simulink model "vC_1ph_MR2"  (Simulink 7.9)
settings: Solver=ode14x  StartTime=0.0  StopTime=20/60  FixedStep=Ts1  RelTol=1e-3
PostLoadFcn:
  | , if any(exist('dsrtsu_mdlpostloadfcn', 'file') == [2, 3, 6]), try dsrtsu_mdlpostloadfcn('Execute', bdroot); catch fprintf('Error in PostLoadFcn (dsrtsu_mdlpostloadfcn) for model "%s":\n %s\n', bdroot, lasterr); end, end,
InitFcn:
  | vC_ini
values from neighbouring files (symbols this model uses):
  C = Cideal+deltaC    (= 4e-05)    [IMC_calculo_limites_thetas.m]    (also in IMC_ini.m; JORGE_controlador_LCL_malha_interna.m; LCL_PAPM.m; R_in_LCL.m)
  excitacao_persistente = 0    [iC_ini.m]    (also in vC_ini.m)
  init_time = 20000/60    (= 333.333333333)    [iC_ini.m]    (also in vC_ini.m)
  L1 = L1ideal+deltaL1    (= 0.002)    [IMC_calculo_limites_thetas.m]    (also in IMC_ini.m; LCL_PAPM.m; R_in_LCL.m; calculo_FTs.m)
  L2 = L2ideal+deltaL2+Lgideal+deltaLg    (= 0.002)    [IMC_calculo_limites_thetas.m]    (also in IMC_ini.m; LCL_PAPM.m; R_in_LCL.m; calculo_FTs.m)
  param_change_time = 20000/60    (= 333.333333333)    [iC_ini.m]    (also in vC_ini.m)
  R1 = R1ideal+deltaR1    (= 1)    [IMC_calculo_limites_thetas.m]    (also in IMC_ini.m; R_in_LCL.m = 0; gera_resultados.m = 0; iC_ini.m = 0)
  R2 = R2ideal+deltaR2+Rgideal+deltaRg    (= 1)    [IMC_calculo_limites_thetas.m]    (also in IMC_ini.m; R_in_LCL.m = 0; gera_resultados.m = 0; iC_ini.m = 0)
  R_init = 10    [iC_ini.m]    (also in vC_ini.m)
  rede_amp = 311    [iC_ini.m]    (also in vC_ini.m)
  ref_amp = 10    [iC_ini.m]    (also in vC_ini.m = 200)
  ref_amp11 = ref_amp/2    (= 5)    [iC_ini.m]    (also in vC_ini.m = 100)
  ref_amp13 = ref_amp/2    (= 5)    [iC_ini.m]    (also in vC_ini.m = 100)
  ref_amp3 = ref_amp/2    (= 5)    [iC_ini.m]    (also in vC_ini.m = 100)
  ref_amp5 = ref_amp/2    (= 5)    [iC_ini.m]    (also in vC_ini.m = 100)
  ref_amp7 = ref_amp/2    (= 5)    [iC_ini.m]    (also in vC_ini.m = 100)
  ref_amp9 = ref_amp/2    (= 5)    [iC_ini.m]    (also in vC_ini.m = 100)
  ref_freq = 2*pi*60    (= 376.991118431)    [iC_ini.m]    (also in vC_ini.m)
  ref_phaseInv_time = 20000/60    (= 333.333333333)    [iC_ini.m]    (also in vC_ini.m)
  ref_step_time = 20000/60    (= 333.333333333)    [iC_ini.m]    (also in vC_ini.m)
  Ts = 0.5    [IMC_calculo_limites_thetas.m]    (also in IMC_datta_ini.m; IMC_ini.m = 8.33333333333e-05; JORGE_controlador_LCL_malha_interna.m = 8.33333333333e-05; LCL_PAPM.m = 8.33333333333e-05)
  Ts1 = Ts/10    (= 8.33333333333e-06)    [iC_ini.m]    (also in vC_ini.m)
  VCC = 400    [iC_ini.m]    (also in vC_ini.m)
libraries: powerlib x15, powerlib_extras x1
settings Model: DSRTSU_INTERNAL_RTI_VER=390  DSRTSU_INTERNAL_RTI_TYPE=rti1103  Creator=dpbernardon  LastModifiedBy=marcelodurgante  BufferReuse=off
settings SolverCC: AutoInsertRateTranBlk=on
settings OptimizationCC: BlockReduction=off  OptimizeBlockIOStorage=off  BufferReuse=off  ExpressionFolding=off  LocalBlockOutputs=off
settings DebuggingCC: FcnCallInpInsideContextMsg=Use local settings  UnconnectedInputMsg=none  UnconnectedOutputMsg=none  UnconnectedLineMsg=none
settings HardwareCC: ProdIntDivRoundTo=Zero  ProdEndianess=BigEndian  ProdHWDeviceType=Generic->Custom  TargetIntDivRoundTo=Zero  TargetEndianess=BigEndian  TargetHWDeviceType=Generic->Custom
settings RTWCC: SystemTargetFile=rti1103.tlc  MakeCommand=make_rti  TemplateMakefile=rti1103.tmf  Description=dSPACE DS1103 Hardware Platform  ProcessScript=rti1103_make_rtw_hook
settings STFCustomTargetCC: CodeReplacementLibrary=ANSI_C  ParMdlRefBuildCompliant=on  GeneratePreprocessorConditionals=Disable all  MatFileLogging=on  SystemTargetFile=rti1103.tlc
settings GRTTargetCC: CompOptLevelCompliant=off  ConcurrentExecutionCompliant=off  CombineOutputUpdateFcns=off  GRTInterface=on  ExtModeMexFile=noextcomm
settings CustomProperty: DataType=RTWOptions_EnumType_C__dSPACE RCPHIL 72_matlab_rti1103_tlc_rti1103_1InitialSimState  Value=RUN
settings EnumStrPairs: String=RUN

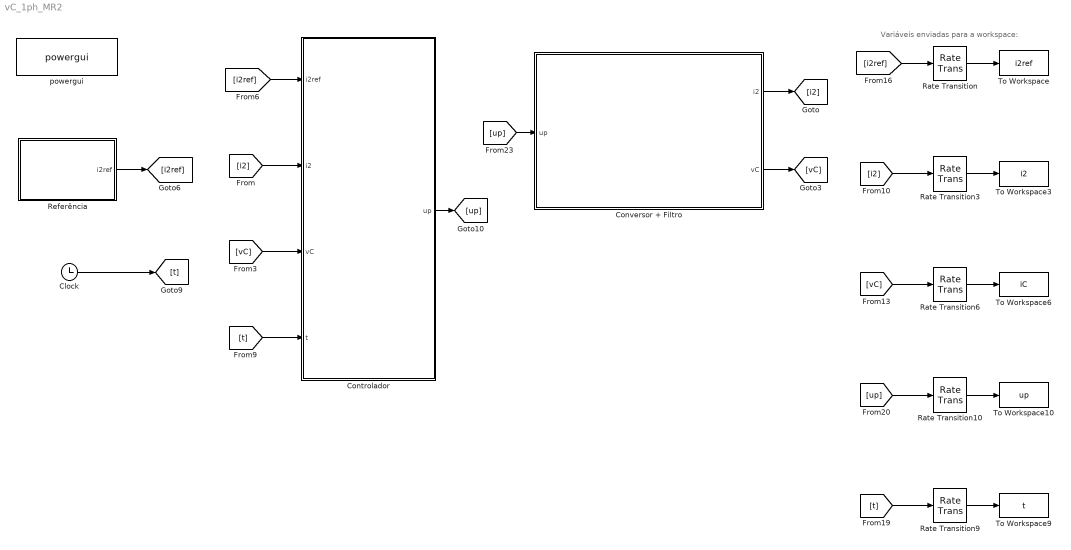
== system vC_1ph_MR2 ==
  note: Variáveis enviadas para a workspace:
  Clock : Clock
  Controlador : Subsystem
  Conversor + Filtro : Subsystem
  Rate Transition{,3,6,9..10} (5 alike) : RateTransition  OutPortSampleTime=Ts1
  Referência : Subsystem
  To Workspace : ToWorkspace  VariableName=i2ref  SampleTime=Ts1
  To Workspace10 : ToWorkspace  VariableName=up  SampleTime=Ts1
  To Workspace3 : ToWorkspace  VariableName=i2  SampleTime=Ts1
  To Workspace6 : ToWorkspace  VariableName=iC  SampleTime=Ts1
  To Workspace9 : ToWorkspace  VariableName=t  SampleTime=Ts1
  powergui : powerlib/powergui  Priority=1  SimulationMode=Discrete  SolverType=Tustin  SampleTime=Ts1  frequency=60  SPID=off  DisableSnubberDevices=off  DisableRonSwitches=off  DisableVfSwitches=off  SwTol=0  Interpol=off  DisplayEquations=off  FunctionMessages=off  frequencyindice=0  Pbase=100e6  ErrMax=1e-4  Iterations=50  UnitsV=kV  UnitsW=MW  echomessages=off  HookPort=off  EnableUseOfTLC=off  x0status=blocks  RestoreLinks=warning  ResistiveCurrentMeasurement=off  Frange=[0:2:500]  Ylog=off  Xlog=on  ShowGrid=off  save=off  variable=ZData  ZoomFFT=off  StartTime=0.0  cycles=1  DisplayStyle=1  fundamental=60  FreqAxis=off  MaxFrequency=1000  frequencyindicesteady=1  RmsSteady=1  display=off  Ts=0  methode=off
  wires:
  Conversor + Filtro/1(i2) -> [i2]
  Conversor + Filtro/2(vC) -> [vC]
  [i2] -> Controlador/2(i2)
  [vC] -> Controlador/3(vC)
  Referência/1(i2ref) -> [i2ref]
  [i2ref] -> Controlador/1(i2ref)
  Clock/1 -> [t]
  [t] -> Controlador/4(t)
  [i2ref] -> Rate Transition/1
  [i2] -> Rate Transition3/1
  [vC] -> Rate Transition6/1
  [t] -> Rate Transition9/1
  Rate Transition/1 -> To Workspace/1
  Rate Transition3/1 -> To Workspace3/1
  Rate Transition6/1 -> To Workspace6/1
  Rate Transition9/1 -> To Workspace9/1
  [up] -> Rate Transition10/1
  Rate Transition10/1 -> To Workspace10/1
  Controlador/1(up) -> [up]
  [up] -> Conversor + Filtro/1(up)

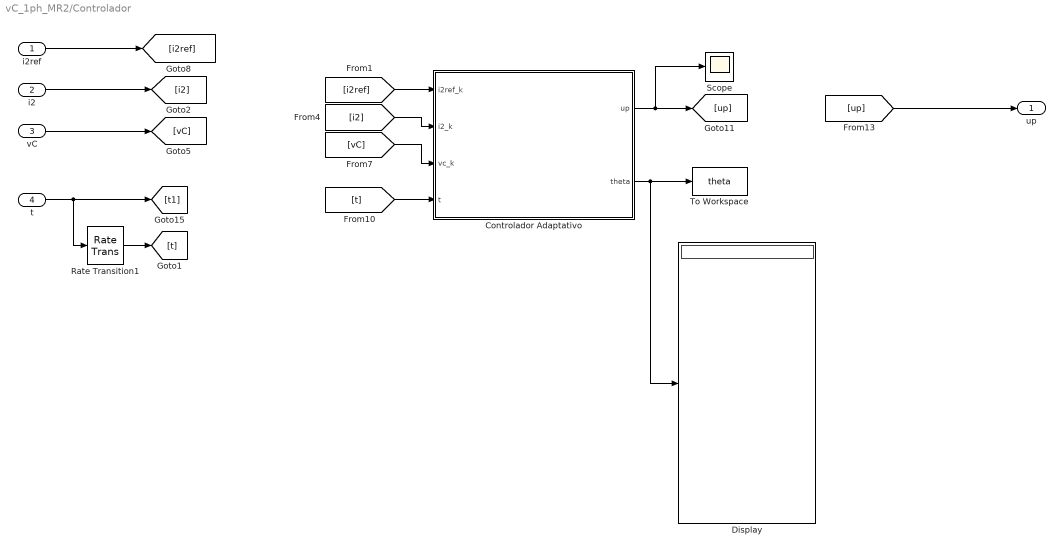
== system vC_1ph_MR2/Controlador ==
  i2ref : Inport
  i2 : Inport  Port=2
  vC : Inport  Port=3
  t : Inport  Port=4
  Controlador Adaptativo : MATLAB Function  TreatAsAtomicUnit=on  SystemSampleTime=Ts
      settings: MinAlgLoopOccurrences=on  RTWSystemCode=Function
  Display : Display
  Rate Transition1 : RateTransition  OutPortSampleTime=Ts
  Scope : Scope
      settings: YMin=-5500  YMax=5000  SaveName=ScopeData4
  To Workspace : ToWorkspace  VariableName=theta  SampleTime=Ts1
  up : Outport
  wires:
  t/1 -> Rate Transition1/1, [t1]
  Rate Transition1/1 -> [t]
  i2/1 -> [i2]
  vC/1 -> [vC]
  [i2ref] -> Controlador Adaptativo/1(i2ref_k)
  [i2] -> Controlador Adaptativo/2(i2_k)
  [vC] -> Controlador Adaptativo/3(vc_k)
  [up] -> up/1
  Controlador Adaptativo/2(theta) -> To Workspace/1, Display/1
  i2ref/1 -> [i2ref]
  Controlador Adaptativo/1(up) -> [up], Scope/1
  [t] -> Controlador Adaptativo/4(t)

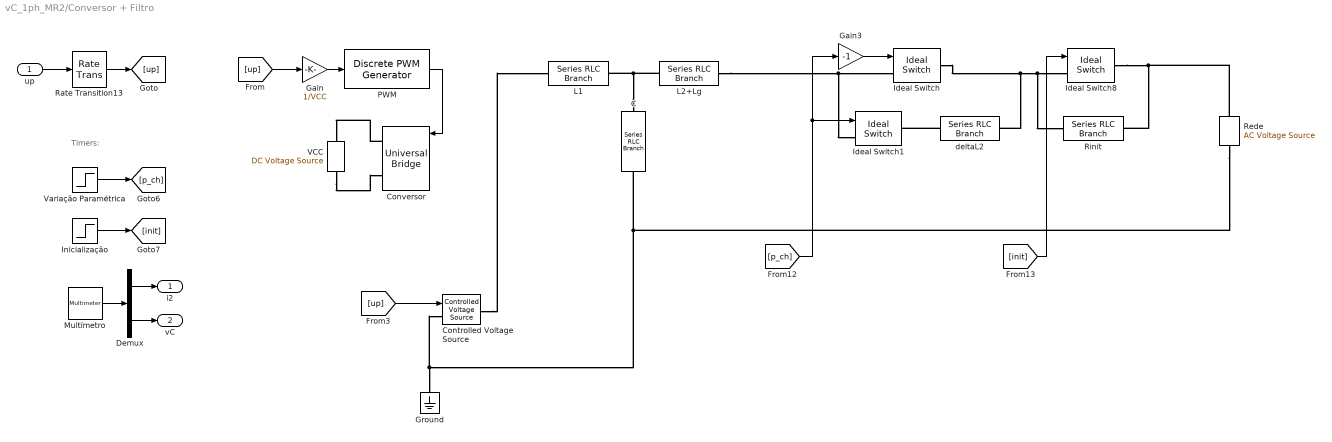
== system vC_1ph_MR2/Conversor + Filtro ==
  note: Timers:
  up : Inport
  C : powerlib/Elements/Series RLC Branch  LConnTagsString=__new0  RConnTagsString=__new0  BranchType=C  Resistance=1  Inductance=1e-3  SetiL0=off  InitialCurrent=0  Capacitance=C  Setx0=off  InitialVoltage=0  Measurements=Branch voltage
  Controlled Voltage Source : powerlib/Electrical Sources/Controlled Voltage Source  Initialize=on  Source_Type=AC  Amplitude=0  Phase=0  Frequency=0  Measurements=None
  Conversor : powerlib/Power Electronics/Universal Bridge  Arms=3  SnubberResistance=1e5  SnubberCapacitance=inf  Device=IGBT / Diodes  Ron=1e-3  Lon=0  ForwardVoltages="[  0  0  ]"  ForwardVoltage=0  GTOparameters=[ 10e-6 , 20e-6 ]  IGBTparameters=[ 1e-6 , 2e-6 ]  Measurements=UAB UBC UCA UDC voltages  Measurements_2=None  converterType=Rectifier
  Demux : Demux  Outputs=2
  Gain : Gain  Gain=1/VCC  SampleTime=Ts1
  Gain3 : Gain  Gain=-1  SampleTime=Ts1
  Ground : powerlib/Elements/Ground  LConnTagsString=a
  Ideal Switch : powerlib/Power Electronics/Ideal Switch  Ron=0.001  Lon=0  IC=1  Rs=1e5  Cs=inf  Measurements=off
  Ideal Switch1 : powerlib/Power Electronics/Ideal Switch  Ron=0.001  Lon=0  IC=0  Rs=1e5  Cs=inf  Measurements=off
  Ideal Switch8 : powerlib/Power Electronics/Ideal Switch  Ron=0.001  Lon=0  IC=1  Rs=1e5  Cs=inf  Measurements=off
  Inicialização : Step  Time=init_time  Before=1  After=0  SampleTime=Ts1
  L1 : powerlib/Elements/Series RLC Branch  LConnTagsString=__new0  RConnTagsString=__new0  BranchType=RL  Resistance=R1  Inductance=L1  SetiL0=off  InitialCurrent=0  Capacitance=1e-6  Setx0=off  InitialVoltage=0  Measurements=None
  L2+Lg : powerlib/Elements/Series RLC Branch  LConnTagsString=__new0  RConnTagsString=__new0  BranchType=RL  Resistance=R2  Inductance=L2  SetiL0=off  InitialCurrent=0  Capacitance=1e-6  Setx0=off  InitialVoltage=0  Measurements=Branch current
  Multímetro : powerlib/Measurements/Multimeter  PhasorSimulation=off  OutputType=Complex  sel=[6 1]  L=6  Gain=[1 1]  yselected={'Ib: Conversor + Filtro/L2+Lg','Ub: Conversor + Filtro/C'};  PSBOutputType=1  PSBequivalent=0  AxesSetting=[0,0.1,-100,100]  Display=0  SavedBlockNames=-11
  PWM : powerlib_extras/Discrete  Control Blocks/Discrete PWM Generator  GeneratorMode="3-arm  bridge (6 pulses)"  Fc=12000  Ts=Ts1  Internal=off  mIndex=0.4  Freq=60  Phase=0
  Rate Transition13 : RateTransition  OutPortSampleTime=Ts1
  Rede : powerlib/Electrical Sources/AC Voltage Source  Amplitude=rede_amp  Phase=0  Frequency=60  SampleTime=0  Measurements=None
  Rinit : powerlib/Elements/Series RLC Branch  LConnTagsString=__new0  RConnTagsString=__new0  BranchType=RL  Resistance=R_init  Inductance=5*L2  SetiL0=off  InitialCurrent=0  Capacitance=1e-6  Setx0=off  InitialVoltage=0  Measurements=None
  VCC : powerlib/Electrical Sources/DC Voltage Source  Amplitude=VCC  Measurements=None
  Variação Paramétrica : Step  Time=param_change_time  Before=-1  SampleTime=Ts1
  deltaL2 : powerlib/Elements/Series RLC Branch  LConnTagsString=__new0  RConnTagsString=__new0  BranchType=RL  Resistance=0  Inductance=5*L2  SetiL0=off  InitialCurrent=0  Capacitance=1e-6  Setx0=off  InitialVoltage=0  Measurements=None
  i2 : Outport
  vC : Outport  Port=2
  wires:
  Gain/1 -> PWM/1
  up/1 -> Rate Transition13/1
  Rate Transition13/1 -> [up]
  PWM/1 -> Conversor/1
  [up] -> Gain/1
  [up] -> Controlled Voltage Source/1
  Multímetro/1 -> Demux/1
  Demux/1 -> i2/1
  Variação Paramétrica/1 -> [p_ch]
  Gain3/1 -> Ideal Switch/1
  [init] -> Ideal Switch8/1
  Inicialização/1 -> [init]
  [p_ch] -> Gain3/1, Ideal Switch1/1
  Demux/2 -> vC/1
  connections:
  Ideal Switch/RConn1 -- deltaL2/RConn1 -- Ideal Switch8/LConn1 -- Rinit/LConn1
  C/LConn1 -- L2+Lg/LConn1 -- L1/RConn1
  Conversor/RConn1 -- VCC/RConn1
  VCC/LConn1 -- Conversor/RConn2
  L2+Lg/RConn1 -- Ideal Switch/LConn1 -- Ideal Switch1/LConn1
  deltaL2/LConn1 -- Ideal Switch1/RConn1
  Controlled Voltage Source/RConn1 -- L1/LConn1
  Rede/RConn1 -- Ideal Switch8/RConn1 -- Rinit/RConn1
  Controlled Voltage Source/LConn1 -- Ground/LConn1 -- C/RConn1 -- Rede/LConn1

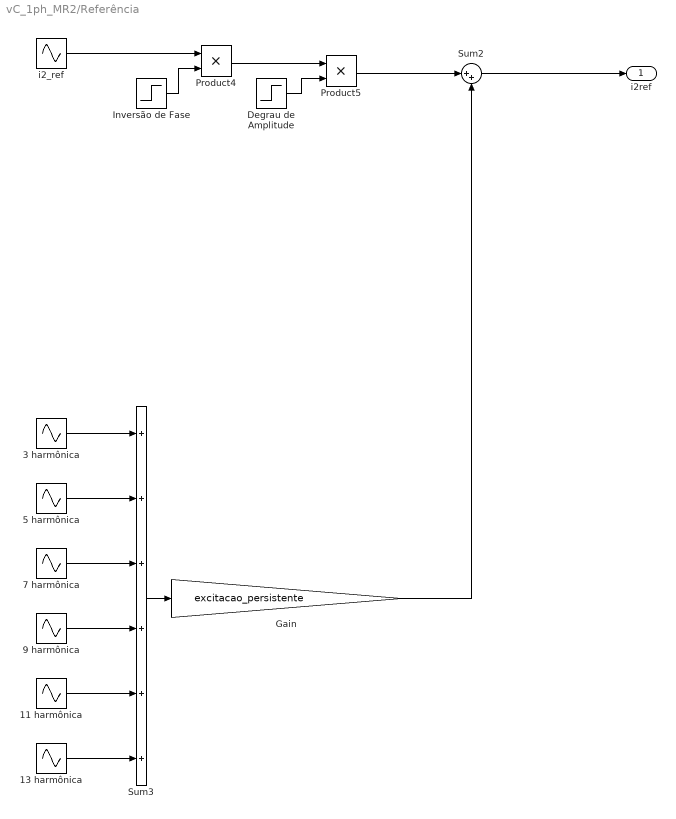
== system vC_1ph_MR2/Referência ==
  11 harmônica : Sin  Amplitude=ref_amp11  Frequency=ref_freq*11  SampleTime=Ts
  13 harmônica : Sin  Amplitude=ref_amp13  Frequency=ref_freq*13  SampleTime=Ts
  3 harmônica : Sin  Amplitude=ref_amp3  Frequency=ref_freq*3  SampleTime=Ts
  5 harmônica : Sin  Amplitude=ref_amp5  Frequency=ref_freq*5  SampleTime=Ts
  7 harmônica : Sin  Amplitude=ref_amp7  Frequency=ref_freq*7  SampleTime=Ts
  9 harmônica : Sin  Amplitude=ref_amp9  Frequency=ref_freq*9  SampleTime=Ts
  Degrau de Amplitude : Step  Time=ref_step_time  Before=1  After=2  SampleTime=Ts
  Gain : Gain  Gain=excitacao_persistente  SampleTime=Ts
  Inversão de Fase : Step  Time=ref_phaseInv_time  Before=1  After=-1  SampleTime=Ts
  Product4 : Product  SampleTime=Ts  RndMeth=Zero
  Product5 : Product  SampleTime=Ts  RndMeth=Zero
  Sum2 : Sum  Inputs=|++
  Sum3 : Sum  Inputs=++++++
  i2_ref : Sin  Amplitude=ref_amp  Frequency=ref_freq  SampleTime=Ts
  i2ref : Outport
  wires:
  Product4/1 -> Product5/1
  Inversão de Fase/1 -> Product4/2
  Degrau de Amplitude/1 -> Product5/2
  i2_ref/1 -> Product4/1
  Product5/1 -> Sum2/1
  Gain/1 -> Sum2/2
  Sum2/1 -> i2ref/1
  3 harmônica/1 -> Sum3/1
  5 harmônica/1 -> Sum3/2
  7 harmônica/1 -> Sum3/3
  9 harmônica/1 -> Sum3/4
  11 harmônica/1 -> Sum3/5
  13 harmônica/1 -> Sum3/6
  Sum3/1 -> Gain/1

== matlab function Controlador/Controlador Adaptativo ==
  data: i2ref_k input double; up output double; i2_k input double; vc_k input double; theta output double; t input double
function [up, theta] = adaptativo( i2ref_k, i2_k, vc_k, t)

%#CODEGEN

%Kp é a multiplicação do ganho do controlador da malha interna(kp), do
%ganho da planta(ki) e do ganho da malha externa(kod)
kp_kd=3;
%Kp=0.156891976007044;
Kp=0.001792815465831;

%polos do modelo de referência:
p1=0.2;
p2=0.2;

km=(1-p1)*(1-p2);

%constantes -> gamaD < (1-gama)*km/kp
%gamaD=0.01;
gamaD=0.0098;
gama=0.99;

delta0=0.99;

%está ligado contra a rede?
rede=1;

%% Variáveis Persistentes e Inicializações

persistent theta_k;
if isempty(theta_k)
    %theta_k=[0.4226; -3.4222; -0.2133; 12.7376; 0; 0];
    theta_k=[0.3258; -2.9077; -0.2815; 13.1402; 0; 0];
end

persistent omega_k;
if isempty(omega_k)
    omega_k=[0; 0; 0; 0; 0; 0];
end

persistent omega_k_1;
if isempty(omega_k_1)
    omega_k_1=[0; 0; 0; 0; 0; 0];
end

persistent omega_k_2;
if isempty(omega_k_2)
    omega_k_2=[0; 0; 0; 0; 0; 0];
end

persistent eta_k_1;
if isempty(eta_k_1)
    eta_k_1=[0; 0; 0; 0; 0; 0];
end

persistent eta_k_2;
if isempty(eta_k_2)
    eta_k_2=[0; 0; 0; 0; 0; 0];
end

persistent i2m_k_1;
if isempty(i2m_k_1)
    i2m_k_1=0;
end

persistent i2m_k_2;
if isempty(i2m_k_2)
    i2m_k_2=0;
end

persistent i2ref_k_1;
if isempty(i2ref_k_1)
    i2ref_k_1=0;
end

persistent i2ref_k_2;
if isempty(i2ref_k_2)
    i2ref_k_2=0;
end

persistent v_k_1;
if isempty(v_k_1)
    v_k_1=0;
end

persistent v_k_2;
if isempty(v_k_2)
    v_k_2=0;
end

persistent rho_k;
if isempty(rho_k)
    rho_k=Kp/km;
end

persistent m2;
if isempty(m2)
    m2=1;
end

persistent vc_k_1;
if isempty(vc_k_1)
    vc_k_1=0;
end

persistent u_k_1;
if isempty(u_k_1)
    u_k_1=0;
end

persistent u_k_2;
if isempty(u_k_2)
    u_k_2=0;
end


%% Cálculos

%Ação de controle
omega_k(3)= i2_k;
omega_k(4)= i2ref_k;

%COM vg
if rede
    omega_k(5)= 311*sin(2*pi*60*t);
    omega_k(6)= 311*cos(2*pi*60*t);
else
%SEM vg
    omega_k(5)= 0;
    omega_k(6)= 0;
end

u_k= theta_k'*omega_k;

%inserindo o controlador proporcional no bloco do adaptativo
up= kp_kd*(u_k - vc_k) - kp_kd*(u_k_1 - vc_k_1);

eta_k= (p1+p2)*eta_k_1 - p1*p2*eta_k_2 + (1-p1)*(1-p2)*omega_k_2;

i2m_k= (p1+p2)*i2m_k_1 - p1*p2*i2m_k_2 + (1-p1)*(1-p2)*i2ref_k_2;

e1_k= i2_k - i2m_k;

v_k= (p1+p2)*v_k_1 - p1*p2*v_k_2 + (1-p1)*(1-p2)*u_k_2;

q_k= theta_k'*eta_k;

e2_k= -v_k+q_k;

ea_k= e1_k+rho_k*e2_k;

m2_k= 0.1*eta_k'*eta_k + e2_k^2 + m2;


%% Atualização

%calcula theta(k+1)
theta_k = theta_k - (gamaD*ea_k/m2_k)*eta_k;
theta = theta_k;

%calcula rho(k+1)
rho_k= rho_k - (gama*ea_k*e2_k)/m2_k;

m2 = delta0*(m2 - 1) + abs(u_k) + abs(i2_k) + 1;

omega_k_2=omega_k_1;
omega_k_1=omega_k;

omega_k(1)=0*omega_k(1) + 1*u_k;
omega_k(2)=0*omega_k(2) + 1*i2_k;

eta_k_2=eta_k_1;
eta_k_1=eta_k;

i2ref_k_2 = i2ref_k_1;
i2ref_k_1 = i2ref_k;

i2m_k_2=i2m_k_1;
i2m_k_1=i2m_k;

v_k_2=v_k_1;
v_k_1=v_k;

u_k_2=u_k_1;
u_k_1=u_k;

vc_k_1=vc_k;

end
